simulink model "drill_model"  (R2022b)
settings: Solver=VariableStepAuto  StartTime=0.0  StopTime=30  RelTol=1e-3
values from neighbouring files (symbols this model uses):
  A = [0 1 -1 0 ... (first row only)    [drill_model_script.m]
  A1 = [A,E*Cd; zeros(length(Ad),length(A)), Ad]    [drill_model_script.m]
  B = [0; 0; 0; beta/(kphi*Te)]    [drill_model_script.m]
  B1 = [B;zeros(length(Ad),1)]    [drill_model_script.m]
  b12 = 2e-4    (= 0.0002)    [drill_model_script.m]
  beta = kphi^2/Ra    (= 0.0240833333333)    [drill_model_script.m]
  C = [0 1 0 0]    [drill_model_script.m]
  C1 = [C,zeros(1,length(Ad))]    [drill_model_script.m]
  c12 = 0.1    [drill_model_script.m]
  J1 = 0.01    [drill_model_script.m]
  J2 = 0.02    [drill_model_script.m]
  kphi = 0.085    [drill_model_script.m]
  L = place(A.',C.',lambda_tilde).'    [drill_model_script.m]
  L1 = place(A1.',C1.',lambda_tilde1).'    [drill_model_script.m]
  Te = La/Ra    (= 0.0333333333333)    [drill_model_script.m]
  xhat1_0 = [0; 100; 100; 0; 1; 0]    [drill_model_script.m]
  xhat_0 = [0; 100; 100; 0]    [drill_model_script.m]
settings Model: Creator=golov  LastModifiedBy=golov

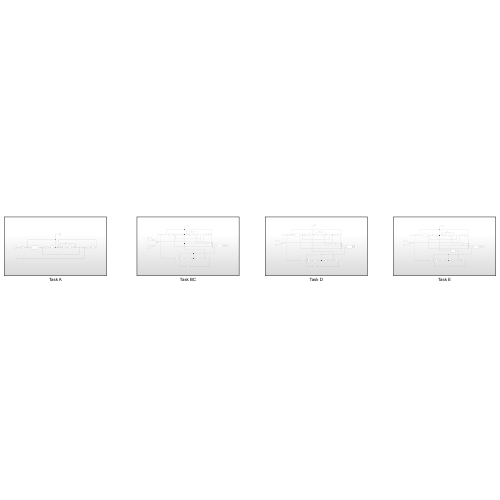
[thumbnail: Simulink's stored preview of the top-level diagram]
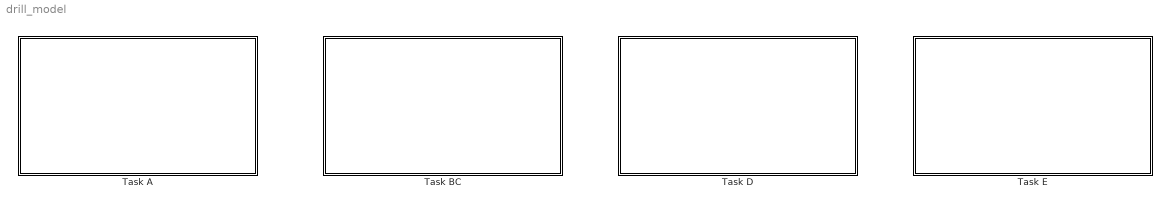
== system drill_model ==
  Task A : Subsystem
  Task BC : Subsystem
  Task D : Subsystem
  Task E : Subsystem

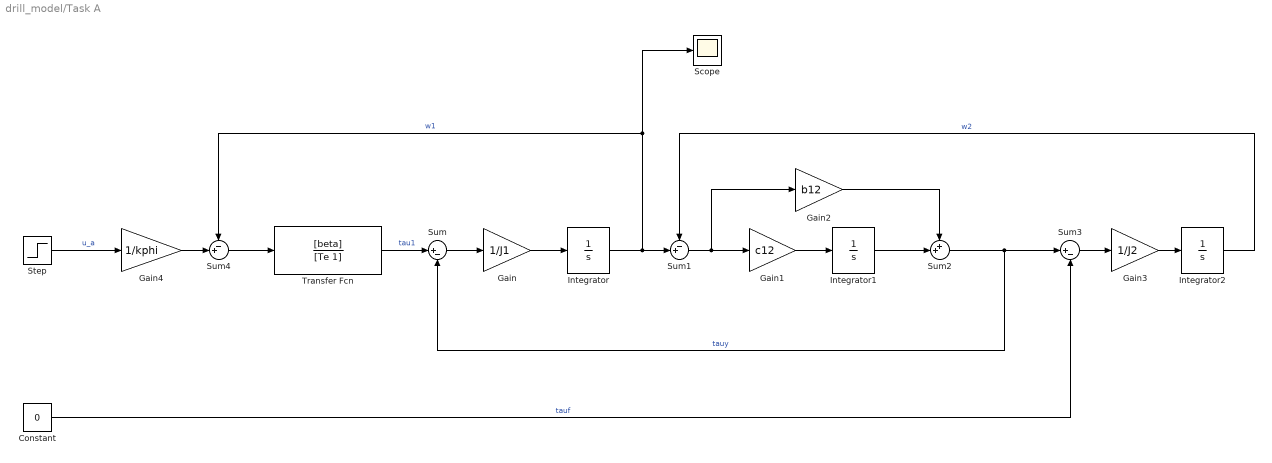
== system drill_model/Task A ==
  Constant : Constant  Value=0
  Gain : Gain  Gain=1/J1
  Gain1 : Gain  Gain=c12
  Gain2 : Gain  Gain=b12
  Gain3 : Gain  Gain=1/J2
  Gain4 : Gain  Gain=1/kphi
  Integrator : Integrator
  Integrator1 : Integrator
  Integrator2 : Integrator
  Scope : Scope
  Step : Step  After=24  SampleTime=0
  Sum : Sum  Inputs=|+-
  Sum1 : Sum  Inputs=-+|
  Sum2 : Sum  Inputs=++|
  Sum3 : Sum  Inputs=|+-
  Sum4 : Sum  Inputs=-+|
  Transfer Fcn : TransferFcn  Numerator=[beta]  Denominator=[Te 1]
  wires:
  Sum4/1 -> Transfer Fcn/1
  Gain4/1 -> Sum4/2
  Integrator/1 -> Scope/1, Sum4/1, Sum1/2  "w1"
  Sum2/1 -> Sum3/1, Sum/2  "tauy"
  Sum/1 -> Gain/1
  Sum1/1 -> Gain2/1, Gain1/1
  Gain1/1 -> Integrator1/1
  Gain2/1 -> Sum2/1
  Integrator2/1 -> Sum1/1  "w2"
  Constant/1 -> Sum3/2  "tauf"
  Gain3/1 -> Integrator2/1
  Integrator1/1 -> Sum2/2
  Step/1 -> Gain4/1  "u_a"
  Transfer Fcn/1 -> Sum/1  "tau1"
  Sum3/1 -> Gain3/1
  Gain/1 -> Integrator/1

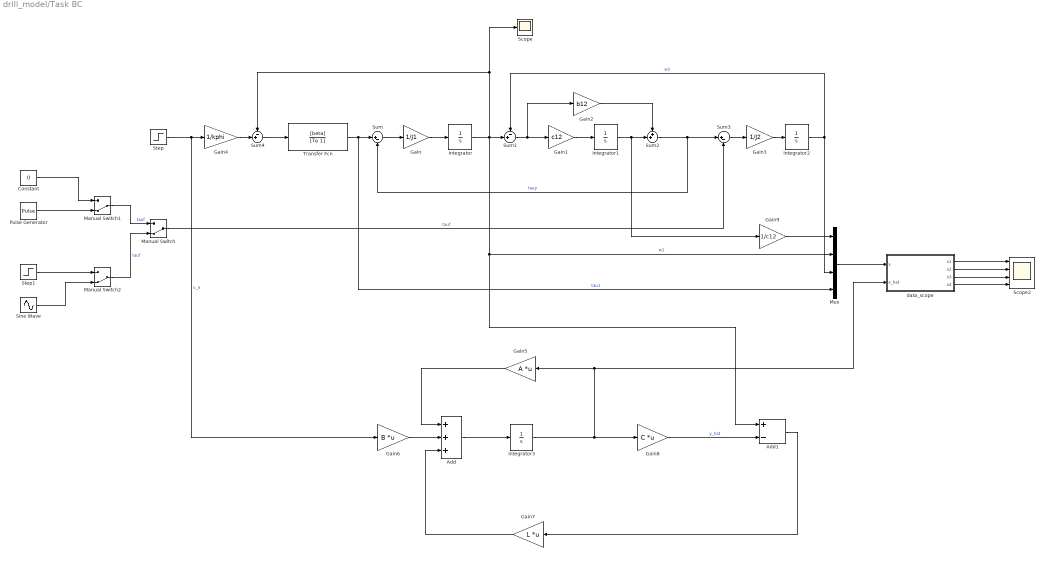
== system drill_model/Task BC ==
  Add : Sum  Inputs=+++
  Add1 : Sum  Inputs=+-
  Constant : Constant  Value=0
  Gain : Gain  Gain=1/J1
  Gain1 : Gain  Gain=c12
  Gain2 : Gain  Gain=b12
  Gain3 : Gain  Gain=1/J2
  Gain4 : Gain  Gain=1/kphi
  Gain5 : Gain  Gain=A  Multiplication=Matrix(K*u)
  Gain6 : Gain  Gain=B  Multiplication=Matrix(K*u)
  Gain7 : Gain  Gain=L  Multiplication=Matrix(K*u)
  Gain8 : Gain  Gain=C  Multiplication=Matrix(K*u)
  Gain9 : Gain  Gain=1/c12
  Integrator : Integrator
  Integrator1 : Integrator
  Integrator2 : Integrator
  Integrator3 : Integrator  InitialCondition=xhat_0
  Manual Switch : ManualSwitch  CurrentSetting=0
  Manual Switch1 : ManualSwitch  CurrentSetting=0
  Manual Switch2 : ManualSwitch  CurrentSetting=0
  Mux : Mux
  Pulse Generator : DiscretePulseGenerator  PulseType=Time based  Period=10
  Scope : Scope
  Scope2 : Scope  NumInputPorts=4
  Sine Wave : Sin  Frequency=0.5  SampleTime=0
  Step : Step  Time=0  After=24  SampleTime=0
  Step1 : Step  Time=10  After=0.2  SampleTime=0
  Sum : Sum  Inputs=|+-
  Sum1 : Sum  Inputs=-+|
  Sum2 : Sum  Inputs=++|
  Sum3 : Sum  Inputs=|+-
  Sum4 : Sum  Inputs=-+|
  Transfer Fcn : TransferFcn  Numerator=[beta]  Denominator=[Te 1]
  data_scope : MATLAB Function  TreatAsAtomicUnit=on
  wires:
  Sum4/1 -> Transfer Fcn/1
  Gain4/1 -> Sum4/2
  Integrator/1 -> Add1/1, Mux/2, Scope/1, Sum4/1, Sum1/2  "w1"
  Sum2/1 -> Sum3/1, Sum/2  "tauy"
  Sum/1 -> Gain/1
  Sum1/1 -> Gain2/1, Gain1/1
  Gain1/1 -> Integrator1/1
  Gain2/1 -> Sum2/1
  Integrator2/1 -> Mux/3, Sum1/1  "w2"
  Manual Switch/1 -> Sum3/2  "tauf"
  Gain3/1 -> Integrator2/1
  Integrator1/1 -> Gain9/1, Sum2/2
  Step/1 -> Gain6/1, Gain4/1  "u_a"
  Transfer Fcn/1 -> Mux/4, Sum/1  "tau1"
  Sum3/1 -> Gain3/1
  Gain/1 -> Integrator/1
  Integrator3/1 -> Gain8/1, data_scope/2(x_hat), Gain5/1
  Gain6/1 -> Add/2
  Add/1 -> Integrator3/1
  Gain5/1 -> Add/1
  Gain7/1 -> Add/3
  Gain8/1 -> Add1/2  "y_hat"
  Add1/1 -> Gain7/1
  data_scope/1(x1) -> Scope2/1
  data_scope/2(x2) -> Scope2/2
  data_scope/3(x3) -> Scope2/3
  data_scope/4(x4) -> Scope2/4
  Mux/1 -> data_scope/1(x)
  Gain9/1 -> Mux/1
  Constant/1 -> Manual Switch1/1
  Manual Switch1/1 -> Manual Switch/1  "tauf"
  Pulse Generator/1 -> Manual Switch1/2
  Step1/1 -> Manual Switch2/1
  Manual Switch2/1 -> Manual Switch/2  "tauf"
  Sine Wave/1 -> Manual Switch2/2

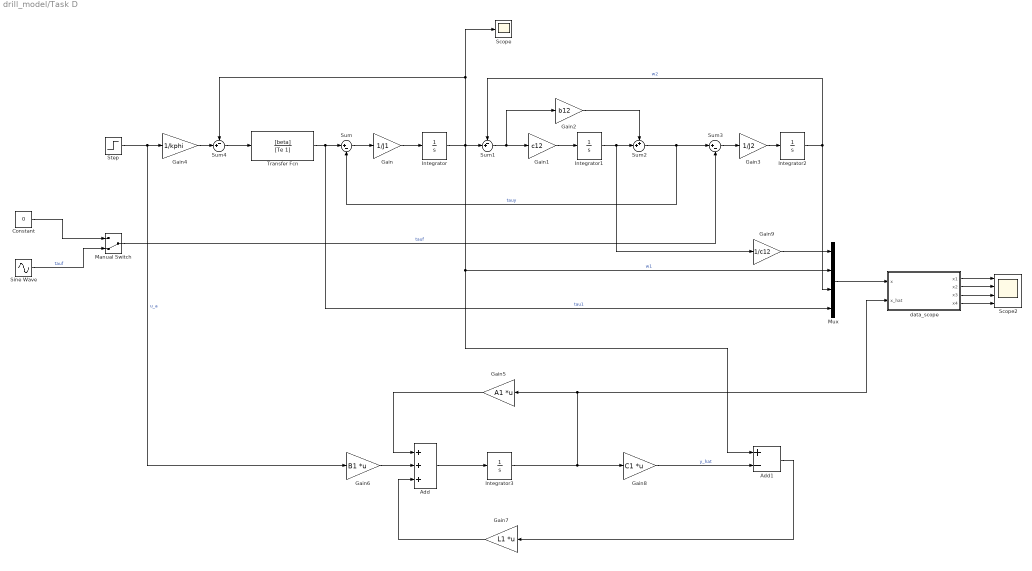
== system drill_model/Task D ==
  Add : Sum  Inputs=+++
  Add1 : Sum  Inputs=+-
  Constant : Constant  Value=0
  Gain : Gain  Gain=1/J1
  Gain1 : Gain  Gain=c12
  Gain2 : Gain  Gain=b12
  Gain3 : Gain  Gain=1/J2
  Gain4 : Gain  Gain=1/kphi
  Gain5 : Gain  Gain=A1  Multiplication=Matrix(K*u)
  Gain6 : Gain  Gain=B1  Multiplication=Matrix(K*u)
  Gain7 : Gain  Gain=L1  Multiplication=Matrix(K*u)
  Gain8 : Gain  Gain=C1  Multiplication=Matrix(K*u)
  Gain9 : Gain  Gain=1/c12
  Integrator : Integrator
  Integrator1 : Integrator
  Integrator2 : Integrator
  Integrator3 : Integrator  InitialCondition=xhat1_0
  Manual Switch : ManualSwitch  CurrentSetting=0
  Mux : Mux
  Scope : Scope
  Scope2 : Scope  NumInputPorts=4
  Sine Wave : Sin  Frequency=0.5  SampleTime=0
  Step : Step  Time=0  After=24  SampleTime=0
  Sum : Sum  Inputs=|+-
  Sum1 : Sum  Inputs=-+|
  Sum2 : Sum  Inputs=++|
  Sum3 : Sum  Inputs=|+-
  Sum4 : Sum  Inputs=-+|
  Transfer Fcn : TransferFcn  Numerator=[beta]  Denominator=[Te 1]
  data_scope : MATLAB Function  TreatAsAtomicUnit=on
  wires:
  Sum4/1 -> Transfer Fcn/1
  Gain4/1 -> Sum4/2
  Integrator/1 -> Add1/1, Mux/2, Scope/1, Sum4/1, Sum1/2  "w1"
  Sum2/1 -> Sum3/1, Sum/2  "tauy"
  Sum/1 -> Gain/1
  Sum1/1 -> Gain2/1, Gain1/1
  Gain1/1 -> Integrator1/1
  Gain2/1 -> Sum2/1
  Integrator2/1 -> Mux/3, Sum1/1  "w2"
  Manual Switch/1 -> Sum3/2  "tauf"
  Gain3/1 -> Integrator2/1
  Integrator1/1 -> Gain9/1, Sum2/2
  Step/1 -> Gain6/1, Gain4/1  "u_a"
  Transfer Fcn/1 -> Mux/4, Sum/1  "tau1"
  Sum3/1 -> Gain3/1
  Gain/1 -> Integrator/1
  Integrator3/1 -> Gain8/1, data_scope/2(x_hat), Gain5/1
  Gain6/1 -> Add/2
  Add/1 -> Integrator3/1
  Gain5/1 -> Add/1
  Gain7/1 -> Add/3
  Gain8/1 -> Add1/2  "y_hat"
  Add1/1 -> Gain7/1
  data_scope/1(x1) -> Scope2/1
  data_scope/2(x2) -> Scope2/2
  data_scope/3(x3) -> Scope2/3
  data_scope/4(x4) -> Scope2/4
  Mux/1 -> data_scope/1(x)
  Gain9/1 -> Mux/1
  Sine Wave/1 -> Manual Switch/2  "tauf"
  Constant/1 -> Manual Switch/1

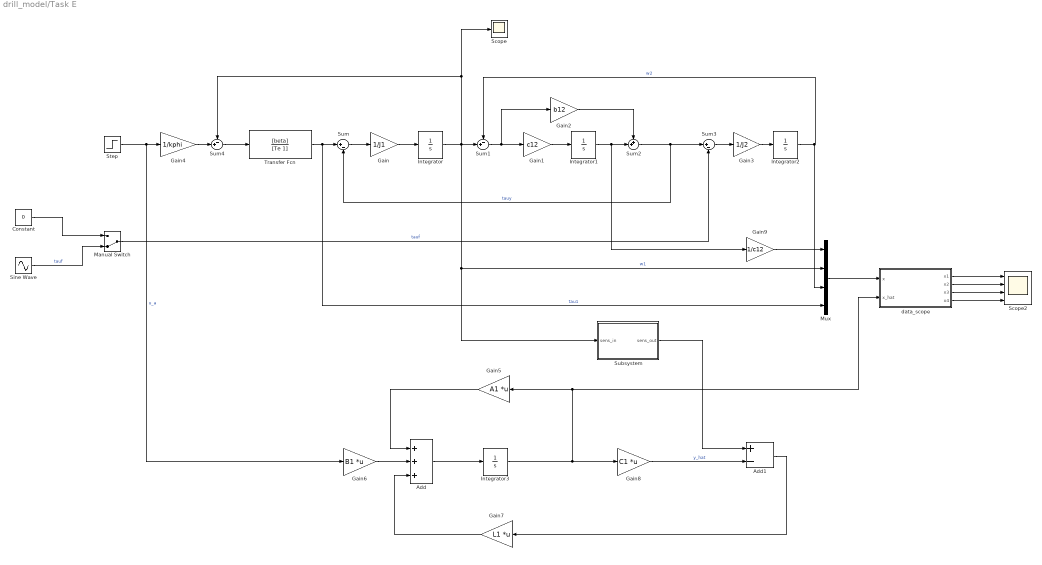
== system drill_model/Task E ==
  Add : Sum  Inputs=+++
  Add1 : Sum  Inputs=+-
  Constant : Constant  Value=0
  Gain : Gain  Gain=1/J1
  Gain1 : Gain  Gain=c12
  Gain2 : Gain  Gain=b12
  Gain3 : Gain  Gain=1/J2
  Gain4 : Gain  Gain=1/kphi
  Gain5 : Gain  Gain=A1  Multiplication=Matrix(K*u)
  Gain6 : Gain  Gain=B1  Multiplication=Matrix(K*u)
  Gain7 : Gain  Gain=L1  Multiplication=Matrix(K*u)
  Gain8 : Gain  Gain=C1  Multiplication=Matrix(K*u)
  Gain9 : Gain  Gain=1/c12
  Integrator : Integrator
  Integrator1 : Integrator
  Integrator2 : Integrator
  Integrator3 : Integrator  InitialCondition=xhat1_0
  Manual Switch : ManualSwitch  CurrentSetting=0
  Mux : Mux
  Scope : Scope
  Scope2 : Scope  NumInputPorts=4
  Sine Wave : Sin  Frequency=0.5  SampleTime=0
  Step : Step  Time=0  After=24  SampleTime=0
  Subsystem : Subsystem
  Sum : Sum  Inputs=|+-
  Sum1 : Sum  Inputs=-+|
  Sum2 : Sum  Inputs=++|
  Sum3 : Sum  Inputs=|+-
  Sum4 : Sum  Inputs=-+|
  Transfer Fcn : TransferFcn  Numerator=[beta]  Denominator=[Te 1]
  data_scope : MATLAB Function  TreatAsAtomicUnit=on
  wires:
  Sum4/1 -> Transfer Fcn/1
  Gain4/1 -> Sum4/2
  Integrator/1 -> Subsystem/1(sens_in), Mux/2, Scope/1, Sum4/1, Sum1/2  "w1"
  Sum2/1 -> Sum3/1, Sum/2  "tauy"
  Sum/1 -> Gain/1
  Sum1/1 -> Gain2/1, Gain1/1
  Gain1/1 -> Integrator1/1
  Gain2/1 -> Sum2/1
  Integrator2/1 -> Mux/3, Sum1/1  "w2"
  Manual Switch/1 -> Sum3/2  "tauf"
  Gain3/1 -> Integrator2/1
  Integrator1/1 -> Gain9/1, Sum2/2
  Step/1 -> Gain6/1, Gain4/1  "u_a"
  Transfer Fcn/1 -> Mux/4, Sum/1  "tau1"
  Sum3/1 -> Gain3/1
  Gain/1 -> Integrator/1
  Integrator3/1 -> Gain8/1, data_scope/2(x_hat), Gain5/1
  Gain6/1 -> Add/2
  Add/1 -> Integrator3/1
  Gain5/1 -> Add/1
  Gain7/1 -> Add/3
  Gain8/1 -> Add1/2  "y_hat"
  Add1/1 -> Gain7/1
  data_scope/1(x1) -> Scope2/1
  data_scope/2(x2) -> Scope2/2
  data_scope/3(x3) -> Scope2/3
  data_scope/4(x4) -> Scope2/4
  Mux/1 -> data_scope/1(x)
  Gain9/1 -> Mux/1
  Sine Wave/1 -> Manual Switch/2  "tauf"
  Constant/1 -> Manual Switch/1
  Subsystem/1(sens_out) -> Add1/1

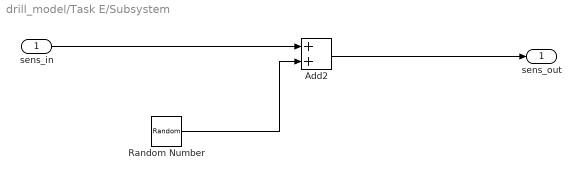
== system drill_model/Task E/Subsystem ==
  sens_in : Inport
  Add2 : Sum
  Random Number : RandomNumber  Variance=10  SampleTime=0.1
  sens_out : Outport
  wires:
  Random Number/1 -> Add2/2
  Add2/1 -> sens_out/1
  sens_in/1 -> Add2/1

== matlab function drill_model/Task D/data_scope ==
  data: x input; x1 output; x_hat input; x2 output; x3 output; x4 output
function [x1, x2, x3, x4] = fcn(x, x_hat)

x1 = [x(1), x_hat(1)];
x2 = [x(2), x_hat(2)];
x3 = [x(3), x_hat(3)];
x4 = [x(4), x_hat(4)];

== matlab function drill_model/Task BC/data_scope ==
  data: x input; x1 output; x_hat input; x2 output; x3 output; x4 output
function [x1, x2, x3, x4] = fcn(x, x_hat)

x1 = [x(1), x_hat(1)];
x2 = [x(2), x_hat(2)];
x3 = [x(3), x_hat(3)];
x4 = [x(4), x_hat(4)];

== matlab function drill_model/Task E/data_scope ==
  data: x input; x1 output; x_hat input; x2 output; x3 output; x4 output
function [x1, x2, x3, x4] = fcn(x, x_hat)

x1 = [x(1), x_hat(1)];
x2 = [x(2), x_hat(2)];
x3 = [x(3), x_hat(3)];
x4 = [x(4), x_hat(4)];
